simulink model "EMI_Resilient_Actuator_Phase2"  (R2026a)
settings: Solver=FixedStepDiscrete  StopTime=1.5  FixedStep=0.001
model workspace (MAT data in the model file):
  EMIActuatorModelSchema.id = 'EMI-ACTUATOR-PARAMETERIZED-V2'
  EMIActuatorModelSchema.kind = 'phase2'
  EMIActuatorModelSchema.plantInputCount = 2
  EMIActuatorModelSchema.supplyLogColumns = 4
settings Model: Creator=adand  LastModifiedBy=adand

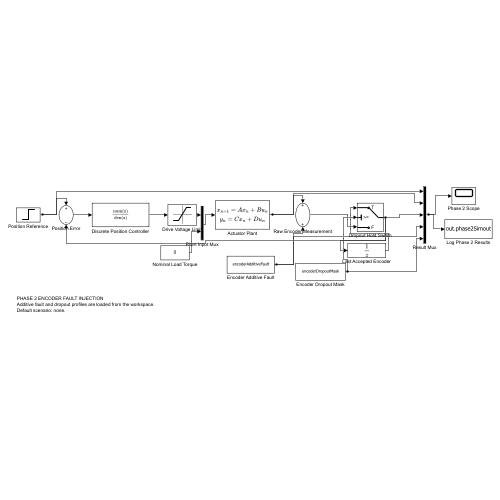
[thumbnail: Simulink's stored preview of the top-level diagram]
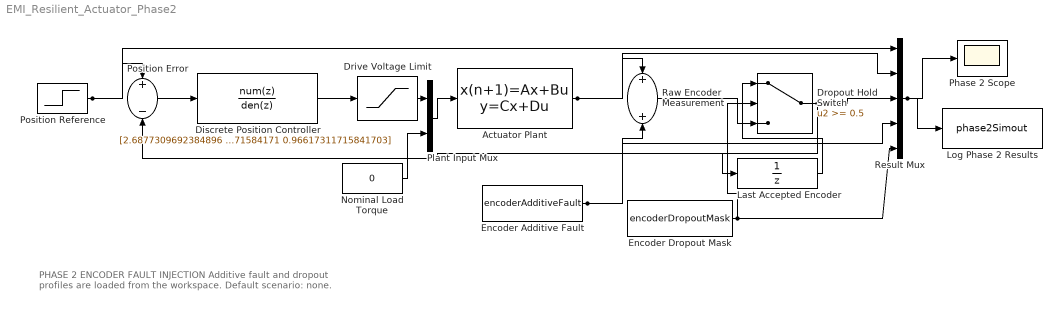
== system EMI_Resilient_Actuator_Phase2 ==
  note: PHASE 2 ENCODER FAULT INJECTION
      | Additive fault and dropout profiles are loaded from the workspace.
      | Default scenario: none.
  Actuator Plant : DiscreteStateSpace  A=[1 0.0009971362516155032 0.00022829831371848575;0 0.99202969645993144 0.42222281027672853;0 -0.025333368616603714 0.61255694572372166]  B=[3.1636509108574085e-05 -0.0033282765581096828;0.09131932548739434 -6.6475750107700211;0.31678125686440572 0.091319325487394326]  C=[1 0 0]  D=[0 0]  InitialCondition=zeros(3,1)  SampleTime=0.001
  Discrete Position Controller : DiscreteTransferFcn  Numerator=[2.6877309692384896 -5.3193946526740499 2.6318328983800279]  Denominator=[1 -1.9661731171584171 0.96617311715841703]  SampleTime=0.001
  Drive Voltage Limit : Saturate  UpperLimit=24  LowerLimit=-24
  Dropout Hold Switch : Switch  Threshold=0.5  SaturateOnIntegerOverflow=off  InputSameDT=off
  Encoder Additive Fault : FromWorkspace  VariableName=encoderAdditiveFault  Interpolate=off  OutputAfterFinalValue=Holding final value
  Encoder Dropout Mask : FromWorkspace  VariableName=encoderDropoutMask  Interpolate=off  OutputAfterFinalValue=Holding final value
  Last Accepted Encoder : UnitDelay  SampleTime=0.001
  Log Phase 2 Results : ToWorkspace  VariableName=phase2Simout  SaveFormat=Structure With Time  SampleTime=-1
  Nominal Load Torque : Constant  Value=0
  Phase 2 Scope : Scope
  Plant Input Mux : Mux  Inputs=2
  Position Error : Sum  Inputs=+-
  Position Reference : Step  Time=0.10000000000000001  FinalValue=0.52359877559829882  SampleTime=0.001
  Raw Encoder Measurement : Sum
  Result Mux : Mux  Inputs=5
  wires:
  Position Reference/1 -> Position Error/1, Result Mux/1
  Position Error/1 -> Discrete Position Controller/1
  Discrete Position Controller/1 -> Drive Voltage Limit/1
  Drive Voltage Limit/1 -> Plant Input Mux/1
  Nominal Load Torque/1 -> Plant Input Mux/2
  Plant Input Mux/1 -> Actuator Plant/1
  Actuator Plant/1 -> Raw Encoder Measurement/1, Result Mux/2
  Encoder Additive Fault/1 -> Raw Encoder Measurement/2, Result Mux/4
  Last Accepted Encoder/1 -> Dropout Hold Switch/1
  Encoder Dropout Mask/1 -> Dropout Hold Switch/2, Result Mux/5
  Raw Encoder Measurement/1 -> Dropout Hold Switch/3
  Dropout Hold Switch/1 -> Last Accepted Encoder/1, Position Error/2, Result Mux/3
  Result Mux/1 -> Phase 2 Scope/1, Log Phase 2 Results/1
